simulink model "image_processing_test"  (R2020b)
settings: Solver=VariableStepAuto  StartTime=0.0  StopTime=10.0  RelTol=1e-3
undefined symbols (not defined in the file): gray, Rec, SDTV
libraries: visiontransforms x2, visionconversions x2, visionstatistics x1, visiontextngfix x1, visionanalysis x1, visionsources x1, parrotlib x1
settings Model: Creator=LIWAN  LastModifiedBy=LIWAN

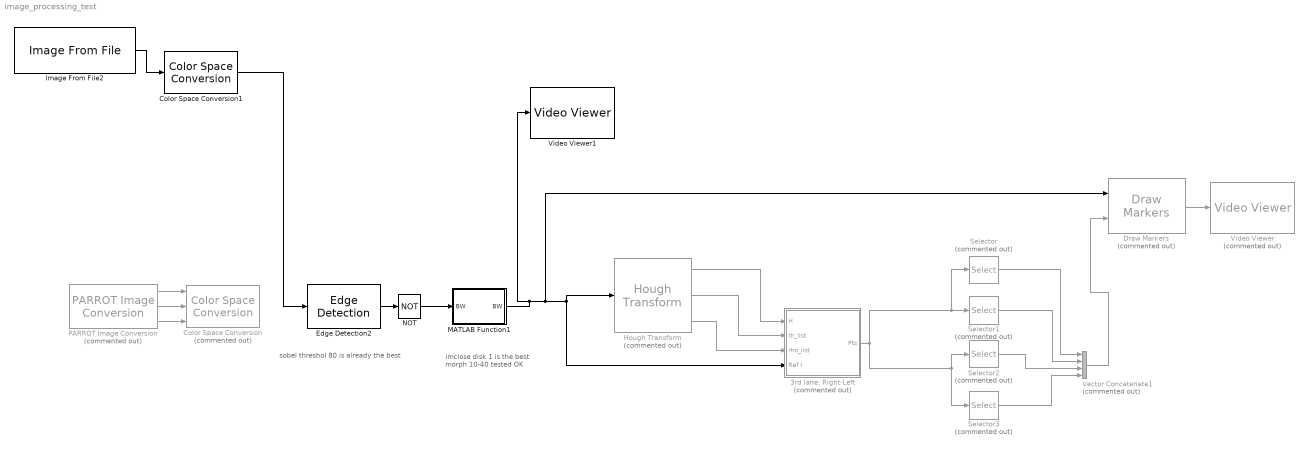
== system image_processing_test ==
  note: sobel threshol 80 is already the best
  note: imclose disk 1 is the best
      | morph 10-40 tested OK
  3rd lane: Right-Left : Subsystem  Commented=on
  Color Space Conversion : visionconversions/Color Space  Conversion  Commented=on  conversion=Obsolete  conversionActive=R'G'B' to intensity  wp_str=D65  rec=Rec. 601 (SDTV)  sys=1125/60/2:1  imagePorts=Separate color signals
  Color Space Conversion1 : visionconversions/Color Space  Conversion  conversion=Obsolete  conversionActive=R'G'B' to intensity  wp_str=D65  rec=Rec. 601 (SDTV)  sys=1125/60/2:1  imagePorts=One multidimensional signal
  Draw Markers : visiontextngfix/Draw Markers  Commented=on  shape=Circle  size=5  fill=off  fillClrSource=Specify via dialog  display=White  intensity=200  color=[200 255 100]  opacity=0.6  viewport=Entire image  antialiasing=off  inType=Obsolete  imagePorts=One multidimensional signal  roundingMode=Floor  overflowMode=off  memoryMode=Specify word length  memoryWordLength=16  memoryFracLength=15  prodOutputMode=Binary point scaling  prodOutputWordLength=32  prodOutputFracLength=14
      settings: SourceProductBaseCode=VP
  Edge Detection2 : visionanalysis/Edge Detection  method=Sobel  outputType=Binary image  userDefinedThreshold=on  thresholdSource=Specify via dialog  threshold=60  thresholdTuning=100  edgeThinning=off  threshold_canny=[0.25 0.75]  autoPercent=70  sigma=1  roundingMode=Floor  overflowMode=off  prodOutputMode=Binary point scaling  prodOutputWordLength=32  prodOutputFracLength=8
      settings: SourceProductBaseCode=VP
  Hough Transform : visiontransforms/Hough Transform  Commented=on  theta_res=pi/180  rho_res=1  out_theta_rho=on  outdtmode=single  roundingMode=Nearest  overflowMode=on  firstCoeffMode=Binary point scaling  firstCoeffWordLength=16  firstCoeffFracLength=14  secondCoeffMode=Binary point scaling  secondCoeffWordLength=32  secondCoeffFracLength=16  prodOutputMode=Binary point scaling  prodOutputWordLength=32  prodOutputFracLength=20  accumMode=Binary point scaling  accumWordLength=32  accumFracLength=20  outputMode=Binary point scaling  outputWordLength=16  outputFracLength=0  memoryMode=Binary point scaling  memoryWordLength=32  memoryFracLength=16
      settings: SourceProductName=Computer Vision Toolbox
  Image From File2 : visionsources/Image From File  Tag=vipblks_nd  FileName=C:\Users\LIWAN\Desktop\sy15\rendu\parrot_gettingstarted\OpenCV_test_project\project\img8.png  Ts=inf  imagePorts=One multidimensional signal  OutPortLabels=R|G|B  ImageDataType=Inherit from input image  sdImageDataType=uint(8)  Signed=on  WordLength=16  FractionLengthMode=User-defined  FractionLength=15
  MATLAB Function1 : MATLAB Function  TreatAsAtomicUnit=on
  NOT : Logic  Operator=NOT  IconShape=distinctive  AllPortsSameDT=off  OutDataTypeStr=boolean
  PARROT Image Conversion : parrotlib/PARROT Image Conversion  Commented=on  ImageFormat=RGB  R=on  Y=on  G=on  U=on  B=on  V=on
      settings: SourceProductName=Simulink Support Package for Parrot Minidrones
  Selector : Selector  Commented=on  NumberOfDimensions=2  InputPortWidth=3  IndexOptions=Index vector (dialog),Index vector (dialog)  Indices=[1],[2 1]  OutputSizes=1,1
  Selector1 : Selector  Commented=on  NumberOfDimensions=2  InputPortWidth=3  IndexOptions=Index vector (dialog),Index vector (dialog)  Indices=[1],[4 3]  OutputSizes=1,1
  Selector2 : Selector  Commented=on  NumberOfDimensions=2  InputPortWidth=3  IndexOptions=Index vector (dialog),Index vector (dialog)  Indices=[2],[2 1]  OutputSizes=1,1
  Selector3 : Selector  Commented=on  NumberOfDimensions=2  InputPortWidth=3  IndexOptions=Index vector (dialog),Index vector (dialog)  Indices=[2],[4 3]  OutputSizes=1,1
  Vector Concatenate1 : Concatenate  Commented=on  NumInputs=4  Mode=Multidimensional array
  Video Viewer : VideoViewer  Commented=on  colormapValue=gray(256)  FigPos=[745.666666666667 589.333333333333 418 304]
  Video Viewer1 : VideoViewer  colormapValue=gray(256)  FigPos=[515.666666666667 631 418 304]
  wires:
  Draw Markers/1 -> Video Viewer/1
  Image From File2/1 -> Color Space Conversion1/1
  PARROT Image Conversion/3 -> Color Space Conversion/3
  Vector Concatenate1/1 -> Draw Markers/2
  Selector1/1 -> Vector Concatenate1/2
  Selector3/1 -> Vector Concatenate1/4
  Edge Detection2/1 -> NOT/1
  MATLAB Function1/1(BW) -> Draw Markers/1, 3rd lane: Right-Left/4(Ref I), Hough Transform/1, Video Viewer1/1
  Hough Transform/3 -> 3rd lane: Right-Left/3(rho_list)
  Selector/1 -> Vector Concatenate1/1
  Hough Transform/2 -> 3rd lane: Right-Left/2(th_list)
  Hough Transform/1 -> 3rd lane: Right-Left/1(H)
  Selector2/1 -> Vector Concatenate1/3
  PARROT Image Conversion/1 -> Color Space Conversion/1
  NOT/1 -> MATLAB Function1/1("BW ")
  3rd lane: Right-Left/1(Pts) -> Selector/1, Selector1/1, Selector3/1, Selector2/1
  PARROT Image Conversion/2 -> Color Space Conversion/2
  Color Space Conversion1/1 -> Edge Detection2/1

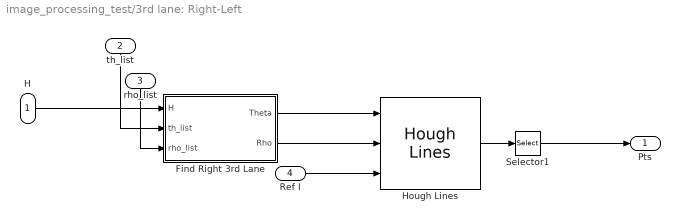
== system image_processing_test/3rd lane: Right-Left ==
  H : Inport
  th_list : Inport  Port=2
  rho_list : Inport  Port=3
  Ref I : Inport  Port=4
  Find Right 3rd Lane : Subsystem
  Hough Lines : visiontransforms/Hough Lines  sineCompMethod=Trigonometric function  thetaRes=pi/180  roundingMode=Nearest  overflowMode=on  firstCoeffMode=Specify word length  firstCoeffWordLength=16  prodOutputMode=Binary point scaling  prodOutputWordLength=32  prodOutputFracLength=16  firstCoeffFracLength=15
      settings: SourceProductName=Computer Vision Toolbox
  Selector1 : Selector  NumberOfDimensions=2  InputPortWidth=3  IndexOptions=Select all,Index vector (dialog)  Indices=[2 1],[2 1 4 3]  OutputSizes=1,1
  Pts : Outport
  wires:
  Ref I/1 -> Hough Lines/3
  Find Right 3rd Lane/2(Rho) -> Hough Lines/2
  Find Right 3rd Lane/1(Theta) -> Hough Lines/1
  H/1 -> Find Right 3rd Lane/1(H)
  th_list/1 -> Find Right 3rd Lane/2(th_list)
  rho_list/1 -> Find Right 3rd Lane/3(rho_list)
  Hough Lines/1 -> Selector1/1
  Selector1/1 -> Pts/1

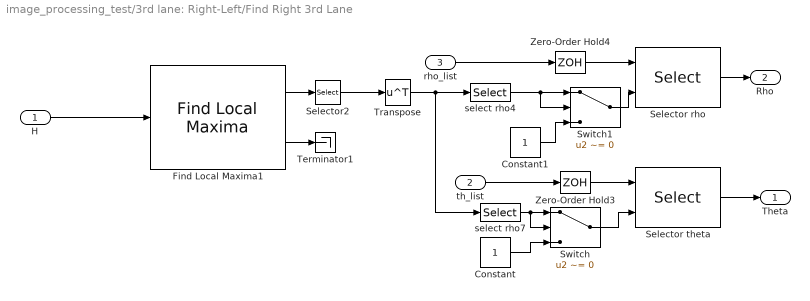
== system image_processing_test/3rd lane: Right-Left/Find Right 3rd Lane ==
  H : Inport
  th_list : Inport  Port=2
  rho_list : Inport  Port=3
  Constant : Constant
  Constant1 : Constant
  Find Local Maxima1 : visionstatistics/Find Local Maxima  num_peaks=2  nhood_size=[9 9]  src_thresh=Obsolete9b  src_thresh_inuse=Specify via dialog  threshold=4  inputIsHough=on  dt_peak=uint16  isOutVarDim=off  dt_count=uint16
      settings: SourceProductName=Computer Vision Toolbox
  Selector rho : Selector  NumberOfDimensions=2  InputPortWidth=3  IndexOptions=Select all,Index vector (port)  Indices=1,2  OutputSizes=1,1
  Selector theta : Selector  NumberOfDimensions=2  InputPortWidth=3  IndexOptions=Select all,Index vector (port)  Indices=1,2  OutputSizes=1,1
  Selector2 : Selector  NumberOfDimensions=2  InputPortWidth=3  IndexOptions=Select all,Index vector (dialog)  Indices=,[2 1]  OutputSizes=1,1
  Switch : Switch  Criteria=u2 ~= 0
  Switch1 : Switch  Criteria=u2 ~= 0
  Terminator1 : Terminator
  Transpose : Math  Operator=transpose  SignedPower=on  SaturateOnIntegerOverflow=on
  Zero-Order Hold3 : ZeroOrderHold  SampleTime=-1
  Zero-Order Hold4 : ZeroOrderHold  SampleTime=-1
  select rho4 : Selector  NumberOfDimensions=2  InputPortWidth=3  IndexOptions=Index vector (dialog),Select all  Indices=1,-1  OutputSizes=1
  select rho7 : Selector  NumberOfDimensions=2  InputPortWidth=3  IndexOptions=Index vector (dialog),Select all  Indices=2,-1  OutputSizes=1
  Theta : Outport
  Rho : Outport  Port=2
  wires:
  Selector theta/1 -> Theta/1
  Find Local Maxima1/2 -> Terminator1/1
  Selector rho/1 -> Rho/1
  H/1 -> Find Local Maxima1/1
  rho_list/1 -> Zero-Order Hold4/1
  Zero-Order Hold4/1 -> Selector rho/1
  th_list/1 -> Zero-Order Hold3/1
  Zero-Order Hold3/1 -> Selector theta/1
  Selector2/1 -> Transpose/1
  Find Local Maxima1/1 -> Selector2/1
  Transpose/1 -> select rho7/1, select rho4/1
  select rho7/1 -> Switch/2, Switch/1
  Switch/1 -> Selector theta/2
  Constant/1 -> Switch/3
  select rho4/1 -> Switch1/1, Switch1/2
  Constant1/1 -> Switch1/3
  Switch1/1 -> Selector rho/2

== matlab function image_processing_test/MATLAB Function1 ==
  data: BW input; BW output
function BW = fcn(BW)
    BW = imclose(BW, strel('disk',2));
    BW = bwmorph(BW, 'skel', 40);
end
